simulink model "Loops10"  (Simulink 8.7)
settings: Solver=ode45  StartTime=0.0  StopTime=10.0  RelTol=1e-3
settings Model: Creator=scaife  LastModifiedBy=bourbouh  ExtModeAutoUpdateStatusClock=off
settings DataIOCC: SignalLoggingSaveFormat=ModelDataLogs  SignalLoggingName=sigsOut
settings OptimizationCC: InitFltsAndDblsToZero=on
settings DebuggingCC: SaveWithParameterizedLinksMsg=none  SignalResolutionControl=TryResolveAllWithWarning  MultiTaskDSMMsg=warning  MultiTaskCondExecSysMsg=none
settings HardwareCC: TargetUnknown=on
settings SFSimCC: SimParseCustomCode=off
settings GRTTargetCC: TargetFcnLib=ansi_tfl_tmw.mat  ModelReferenceCompliant=off  GeneratePreprocessorConditionals=Use local settings  CombineOutputUpdateFcns=off  MatFileLogging=off  GRTInterface=on

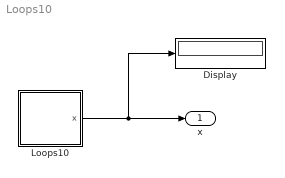
== system Loops10 ==
  Display : Display
  Loops10 : Stateflow chart  TreatAsAtomicUnit=on
  x : Outport
  wires:
  Loops10/1(x) -> x/1, Display/1

== stateflow chart Loops10 ==
  state A
  state B
  state C
  (default) -> A
  (junction 7) -> A [order 3]
  (junction 8) -> C [order 1] : [x==1]
  (junction 7) -> (junction 8) [order 1] : [x==0||x==1]
  A -> (junction 7) : {x=0}
  C -> (junction 8) : {x=2}
  (junction 8) -> (junction 7) [order 3]
  (junction 7) -> (junction 9) [order 2] : [x==2]
  (junction 9) -> (junction 7) [order 3]
  (junction 8) -> (junction 9) [order 2] : [x==0]
  (junction 9) -> (junction 8) [order 1] : [x==3]
  (junction 9) -> B [order 2] : [x==0||x==2]
  B -> (junction 9) : {x++}
  data: x output int32
